simulink model "Robot"  (R2024b)
settings: Solver=ode4  StartTime=0.0  StopTime=inf  FixedStep=1/500  RelTol=1e-3  EnableMultiTasking=on
model workspace (MAT data in the model file):
  SL_ROS_VariableLengthArrays_MaxSizes.CommonInfo.ArrayTruncateAction = 'EmitWarning'
  SL_ROS_VariableLengthArrays_MaxSizes.MsgTypeMap = containers.Map
  SL_ROS_VariableLengthArrays_MaxSizes.MsgTypeMap.serialization.keys = {'trajectory_msgs/JointTrajectoryPoint'}
  SL_ROS_VariableLengthArrays_MaxSizes.MsgTypeMap.serialization.values{1}(1).PropertyName = 'accelerations'
  SL_ROS_VariableLengthArrays_MaxSizes.MsgTypeMap.serialization.values{1}(1).DataType = 'double'
  SL_ROS_VariableLengthArrays_MaxSizes.MsgTypeMap.serialization.values{1}(1).MaxLength = 4
  SL_ROS_VariableLengthArrays_MaxSizes.MsgTypeMap.serialization.values{1}(2).PropertyName = 'effort'
  SL_ROS_VariableLengthArrays_MaxSizes.MsgTypeMap.serialization.values{1}(2).DataType = 'double'
  SL_ROS_VariableLengthArrays_MaxSizes.MsgTypeMap.serialization.values{1}(2).MaxLength = 4
  SL_ROS_VariableLengthArrays_MaxSizes.MsgTypeMap.serialization.values{1}(3).PropertyName = 'positions'
  SL_ROS_VariableLengthArrays_MaxSizes.MsgTypeMap.serialization.values{1}(3).DataType = 'double'
  SL_ROS_VariableLengthArrays_MaxSizes.MsgTypeMap.serialization.values{1}(3).MaxLength = 5
  SL_ROS_VariableLengthArrays_MaxSizes.MsgTypeMap.serialization.values{1}(4).PropertyName = 'velocities'
  SL_ROS_VariableLengthArrays_MaxSizes.MsgTypeMap.serialization.values{1}(4).DataType = 'double'
  SL_ROS_VariableLengthArrays_MaxSizes.MsgTypeMap.serialization.values{1}(4).MaxLength = 4
  SL_ROS_VariableLengthArrays_MaxSizes.MsgTypeMap.serialization.uniformity = 0
  SL_ROS_VariableLengthArrays_MaxSizes.MsgTypeMap.serialization.keyType = 'char'
  SL_ROS_VariableLengthArrays_MaxSizes.MsgTypeMap.serialization.valueType = 'any'
undefined symbols (not defined in the file or in its folder): HIL, positions, positions_SL_Info
libraries: quarc_library x6, ros2lib x3
settings Model: ExtModeTrigDuration=10000  Creator=fvranes  LastModifiedBy=924287296
settings SolverCC: AlgebraicLoopSolver=TrustRegion  PositivePriorityOrder=on
settings DataIOCC: ReturnWorkspaceOutputs=off
settings OptimizationCC: DefaultParameterBehavior=Inlined  EnhancedBackFolding=on  PassReuseOutputArgsThreshold=0  MaxStackSize=64  OptimizeBlockOrder=speed  DifferentSizesBufferReuse=on  OptimizationCustomize=off
settings DebuggingCC: UnderspecifiedInitializationDetection=Classic  MergeDetectMultiDrivingBlocksExec=none  ParameterTunabilityLossMsg=error  UnconnectedInputMsg=warning  UnconnectedOutputMsg=warning  UnconnectedLineMsg=warning
settings ModelReferenceCC: EnableRefExpFcnMdlSchedulingChecks=on  PropagateSignalLabelsOutOfModel=off
settings SFSimCC: MATLABDynamicMemAlloc=off  CustomCodeUndefinedFunction=UseInterfaceOnly
settings RTWCC: Description=QUARC Win64 Target Using Toolchain  SystemTargetFile=quarc_win64.tlc  PackageGeneratedCodeAndArtifacts=on  TemplateMakefile=sldrt.tmf  Toolchain=QUARC win64 | nmake (64-bit Windows)  TargetLang=C++  GPUComputeCapability=3.5
settings RTWCC: CustomInclude=|
  | "Robot_ert_rtw"
  | "C:\Program Files\MATLAB\R2024b\sys\ros2\win64\ros2\include"
  | "C:\Program Files\MATLAB\R2024b\sys\ros2\win64\ros2\include\actionlib_msgs"
  | "C:\Program Files\MATLAB\R2024b\sys\ros2\win64\ros2\include\action_msgs"
  | "C:\Program Files\MATLAB\R2024b\sys\ros2\win64\ros2\include\action_tutorials_interfaces"
  | "C:\Program Files\MATLAB\R2024b\sys\ros2\win64\ros2\include\ament_index_cpp"
  | "C:\Program Files\MATLAB\R2024b\sys\ros2\win64\ros2\include\builtin_interfaces"
  | "C:\Program Files\MATLAB\R2024b\sys\ros2\win64\ros2\include\class_loader"
  | "C:\Program Files\MATLAB\R2024b\sys\ros2\win64\ros2\include\composition_interfaces"
  | "C:\Program Files\MATLAB\R2024b\sys\ros2\win64\ros2\include\console_bridge_vendor"
  | "C:\Program Files\MATLAB\R2024b\sys\ros2\win64\ros2\include\control_msgs"
  | "C:\Program Files\MATLAB\R2024b\sys\ros2\win64\ros2\include\dds"
  | "C:\Program Files\MATLAB\R2024b\sys\ros2\win64\ros2\include\ddsc"
  | "C:\Program Files\MATLAB\R2024b\sys\ros2\win64\ros2\include\diagnostic_msgs"
  | "C:\Program Files\MATLAB\R2024b\sys\ros2\win64\ros2\include\example_interfaces"
  | "C:\Program Files\MATLAB\R2024b\sys\ros2\win64\ros2\include\fastcdr"
  | "C:\Program Files\MATLAB\R2024b\sys\ros2\win64\ros2\include\fastdds"
  | "C:\Program Files\MATLAB\R2024b\sys\ros2\win64\ros2\include\fastrtps"
  | "C:\Program Files\MATLAB\R2024b\sys\ros2\win64\ros2\include\foonathan_memory"
  | "C:\Program Files\MATLAB\R2024b\sys\ros2\win64\ros2\include\geometry_msgs"
  | "C:\Program Files\MATLAB\R2024b\sys\ros2\win64\ros2\include\idl"
  | "C:\Program Files\MATLAB\R2024b\sys\ros2\win64\ros2\include\idlc"
  | "C:\Program Files\MATLAB\R2024b\sys\ros2\win64\ros2\include\keyboard_handler"
  | "C:\Program Files\MATLAB\R2024b\sys\ros2\win64\ros2\include\libstatistics_collector"
  | "C:\Program Files\MATLAB\R2024b\sys\ros2\win64\ros2\include\libyaml_vendor"
  | "C:\Program Files\MATLAB\R2024b\sys\ros2\win64\ros2\include\lifecycle_msgs"
  | "C:\Program Files\MATLAB\R2024b\sys\ros2\win64\ros2\include\logging_demo"
  | "C:\Program Files\MATLAB\R2024b\sys\ros2\win64\ros2\include\map_msgs"
  | "C:\Program Files\MATLAB\R2024b\sys\ros2\win64\ros2\include\mcap_vendor"
  | "C:\Program Files\MATLAB\R2024b\sys\ros2\win64\ros2\include\message_filters"
  | "C:\Program Files\MATLAB\R2024b\sys\ros2\win64\ros2\include\mimick"
  | "C:\Program Files\MATLAB\R2024b\sys\ros2\win64\ros2\include\moodycamel"
  | "C:\Program Files\MATLAB\R2024b\sys\ros2\win64\ros2\include\nav_msgs"
  | "C:\Program Files\MATLAB\R2024b\sys\ros2\win64\ros2\include\octomap_msgs"
  | "C:\Program Files\MATLAB\R2024b\sys\ros2\win64\ros2\include\pendulum_msgs"
  | "C:\Program Files\MATLAB\R2024b\sys\ros2\win64\ros2\include\pluginlib"
  | "C:\Program Files\MATLAB\R2024b\sys\ros2\win64\ros2\include\pybind11_vendor"
  | "C:\Program Files\MATLAB\R2024b\sys\ros2\win64\ros2\include\rcl"
  | "C:\Program Files\MATLAB\R2024b\sys\ros2\win64\ros2\include\rclcpp"
  | "C:\Program Files\MATLAB\R2024b\sys\ros2\win64\ros2\include\rclcpp_action"
  | "C:\Program Files\MATLAB\R2024b\sys\ros2\win64\ros2\include\rclcpp_components"
  | "C:\Program Files\MATLAB\R2024b\sys\ros2\win64\ros2\include\rclcpp_lifecycle"
  | "C:\Program Files\MATLAB\R2024b\sys\ros2\win64\ros2\include\rcl_action"
  | "C:\Program Files\MATLAB\R2024b\sys\ros2\win64\ros2\include\rcl_interfaces"
  | "C:\Program Files\MATLAB\R2024b\sys\ros2\win64\ros2\include\rcl_lifecycle"
  | "C:\Program Files\MATLAB\R2024b\sys\ros2\win64\ros2\include\rcl_logging_interface"
  | "C:\Program Files\MATLAB\R2024b\sys\ros2\win64\ros2\include\rcl_yaml_param_parser"
  | "C:\Program Files\MATLAB\R2024b\sys\ros2\win64\ros2\include\rcpputils"
  | "C:\Program Files\MATLAB\R2024b\sys\ros2\win64\ros2\include\rcutils"
  | "C:\Program Files\MATLAB\R2024b\sys\ros2\win64\ros2\include\rmw"
  | "C:\Program Files\MATLAB\R2024b\sys\ros2\win64\ros2\include\rmw_connextdds"
  | "C:\Program Files\MATLAB\R2024b\sys\ros2\win64\ros2\include\rmw_dds_common"
  | "C:\Program Files\MATLAB\R2024b\sys\ros2\win64\ros2\include\rmw_fastrtps_cpp"
  | "C:\Program Files\MATLAB\R2024b\sys\ros2\win64\ros2\include\rmw_fastrtps_dynamic_cpp"
  | "C:\Program Files\MATLAB\R2024b\sys\ros2\win64\ros2\include\rmw_fastrtps_shared_cpp"
  | "C:\Program Files\MATLAB\R2024b\sys\ros2\win64\ros2\include\ros2cli_test_interfaces"
  | "C:\Program Files\MATLAB\R2024b\sys\ros2\win64\ros2\include\rosbag2_compression"
  | "C:\Program Files\MATLAB\R2024b\sys\ros2\win64\ros2\include\rosbag2_compression_zstd"
  | "C:\Program Files\MATLAB\R2024b\sys\ros2\win64\ros2\include\rosbag2_cpp"
  | "C:\Program Files\MATLAB\R2024b\sys\ros2\win64\ros2\include\rosbag2_interfaces"
  | "C:\Program Files\MATLAB\R2024b\sys\ros2\win64\ros2\include\rosbag2_storage"
  | "C:\Program Files\MATLAB\R2024b\sys\ros2\win64\ros2\include\rosbag2_storage_default_plugins"
  | "C:\Program Files\MATLAB\R2024b\sys\ros2\win64\ros2\include\rosbag2_test_common"
  | "C:\Program Files\MATLAB\R2024b\sys\ros2\win64\ros2\include\rosbag2_transport"
  | "C:\Program Files\MATLAB\R2024b\sys\ros2\win64\ros2\include\rosgraph_msgs"
  | "C:\Program Files\MATLAB\R2024b\sys\ros2\win64\ros2\include\rosidl_runtime_c"
  | "C:\Program Files\MATLAB\R2024b\sys\ros2\win64\ros2\include\rosidl_runtime_cpp"
  | "C:\Program Files\MATLAB\R2024b\sys\ros2\win64\ros2\include\rosidl_typesupport_c"
  | "C:\Program Files\MATLAB\R2024b\sys\ros2\win64\ros2\include\rosidl_typesupport_cpp"
  | "C:\Program Files\MATLAB\R2024b\sys\ros2\win64\ros2\include\rosidl_typesupport_fastrtps_c"
  | "C:\Program Files\MATLAB\R2024b\sys\ros2\win64\ros2\include\rosidl_typesupport_fastrtps_cpp"
  | "C:\Program Files\MATLAB\R2024b\sys\ros2\win64\ros2\include\rosidl_typesupport_interface"
  | "C:\Program Files\MATLAB\R2024b\sys\ros2\win64\ros2\include\rosidl_typesupport_introspection_c"
  | "C:\Program Files\MATLAB\R2024b\sys\ros2\win64\ros2\include\rosidl_typesupport_introspection_cpp"
  | "C:\Program Files\MATLAB\R2024b\sys\ros2\win64\ros2\include\sensor_msgs"
  | "C:\Program Files\MATLAB\R2024b\sys\ros2\win64\ros2\include\shape_msgs"
  | "C:\Program Files\MATLAB\R2024b\sys\ros2\win64\ros2\include\spdlog"
  | "C:\Program Files\MATLAB\R2024b\sys\ros2\win64\ros2\include\statistics_msgs"
  | "C:\Program Files\MATLAB\R2024b\sys\ros2\win64\ros2\include\std_msgs"
  | "C:\Program Files\MATLAB\R2024b\sys\ros2\win64\ros2\include\std_srvs"
  | "C:\Program Files\MATLAB\R2024b\sys\ros2\win64\ros2\include\stereo_msgs"
  | "C:\Program Files\MATLAB\R2024b\sys\ros2\win64\ros2\include\test_msgs"
  | "C:\Program Files\MATLAB\R2024b\sys\ros2\win64\ros2\include\tf2"
  | "C:\Program Files\MATLAB\R2024b\sys\ros2\win64\ros2\include\tf2_msgs"
  | "C:\Program Files\MATLAB\R2024b\sys\ros2\win64\ros2\include\tf2_ros"
  | "C:\Program Files\MATLAB\R2024b\sys\ros2\win64\ros2\include\tracetools"
  | "C:\Program Files\MATLAB\R2024b\sys\ros2\win64\ros2\include\trajectory_msgs"
  | "C:\Program Files\MATLAB\R2024b\sys\ros2\win64\ros2\include\unique_identifier_msgs"
  | "C:\Program Files\MATLAB\R2024b\sys\ros2\win64\ros2\include\visualization_msgs"
  | "C:\Program Files\MATLAB\R2024b\toolbox\ros\slros2\src"
settings CodeAppCC: ForceParamTrailComments=on  MaxIdLength=95  OperatorAnnotations=on
settings STFCustomTargetCC: TargetLangStandard=C++20 (ISO)  ConcurrentExecutionCompliant=on  GRTInterface=on  UseToolchainInfoCompliant=on  SystemTargetFile=quarc_win64.tlc
settings GRTTargetCC: TargetLangStandard=C++20 (ISO)  ParMdlRefBuildCompliant=off  CompOptLevelCompliant=off  CombineOutputUpdateFcns=off  MatFileLogging=off  CPPClassGenCompliant=off  GRTInterface=on  ExtMode=on  ExtModeMexFile=quarc_comm

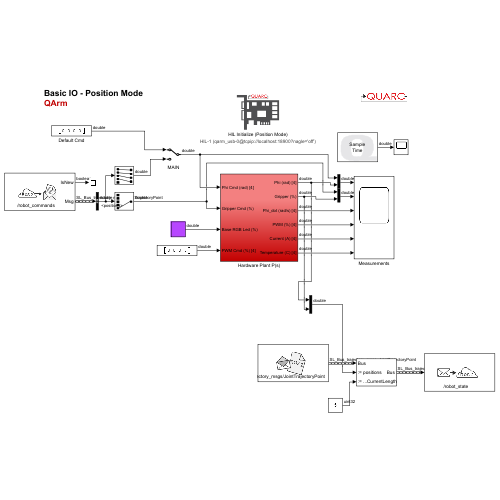
[thumbnail: Simulink's stored preview of the top-level diagram]
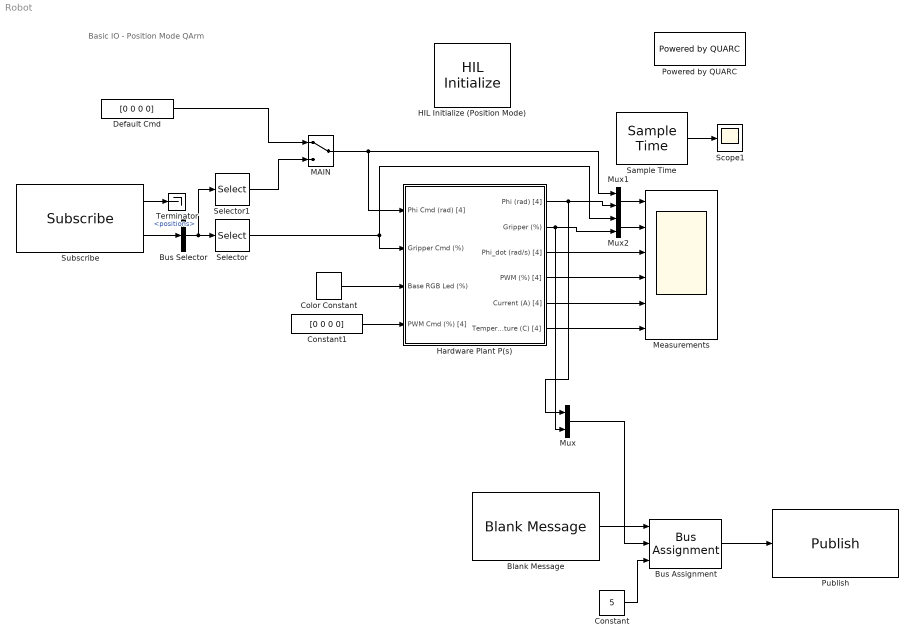
== system Robot ==
  note: Basic IO - Position Mode
      | QArm
  Blank Message : ros2lib/Blank Message  messageClass=Message  entityType=trajectory_msgs/JointTrajectoryPoint  messageType=trajectory_msgs/JointTrajectoryPoint  SampleTime=inf
  Bus Assignment : BusAssignment  AssignedSignals=positions,positions_SL_Info.CurrentLength
  Bus Selector : BusSelector  OutputSignals=positions
  Color Constant : quarc_library/Sources/Signals/Color Constant  color=[0.71765 0.27451 1]
      settings: SourceProductName=QUARC Targets
  Constant : Constant  Value=5  OutDataTypeStr=uint32
  Constant1 : Constant  Value=[0 0 0 0]
  Default Cmd : Constant  Value=[0 0 0 0]
  HIL Initialize (Position Mode) : quarc_library/Data Acquisition/Generic/Configuration/HIL Initialize  object_name=HIL-1  board_type=qarm_usb  board_number=0@tcpip://localhost:18900?nagle='off'  board_options=j0_mode=0;j1_mode=0;j2_mode=0;j3_mode=0;gripper_mode=0;  exclusive=off  active=on  hardware_clocks=[0]  clock_modes=[]  initial_clock_frequencies=[]  set_clock_params_at_start=off  set_clock_params_at_switch_in=off  set_clock_frequencies_at_start=off  set_clock_frequencies_at_switch_in=off  analog_input_channels=[5:9]  analog_input_configurations=[]  analog_input_maximums=[]  analog_input_minimums=[]  set_analog_input_params_at_start=off  set_analog_input_params_at_switch_in=off  analog_output_channels=[]  analog_output_maximums=inf  analog_output_minimums=-inf  initial_analog_outputs=[0]  final_analog_outputs=[0]  watchdog_analog_outputs=[]  set_analog_output_params_at_start=off  set_analog_output_params_at_switch_in=off  set_analog_outputs_at_start=off  set_analog_outputs_at_switch_in=off  set_analog_outputs_at_terminate=off  set_analog_outputs_at_switch_out=off  set_analog_outputs_on_watchdog=off  digital_input_channels=[]  digital_output_channels=[]  digital_output_configuration=[]  initial_digital_outputs=[0]  final_digital_outputs=[0]  watchdog_digital_outputs=[0]  set_digital_output_params_at_start=off  set_digital_output_params_at_switch_in=off  set_digital_outputs_at_start=off  set_digital_outputs_at_switch_in=off  set_digital_outputs_at_terminate=off  set_digital_outputs_at_switch_out=off  set_digital_outputs_on_watchdog=off  encoder_channels=[]  quadrature=[]  encoder_filter_frequency=[]  initial_encoder_counts=[]  set_encoder_params_at_start=off  set_encoder_params_at_switch_in=off  set_encoder_counts_at_start=off  set_encoder_counts_at_switch_in=off  pwm_channels=[]  pwm_modes=[]  pwm_frequency=[]  pwm_configuration=[]  pwm_alignment=[]  pwm_polarity=[]  pwm_leading_deadband=[]  pwm_trailing_deadband=[]  initial_pwm_outputs=[]  final_pwm_outputs=[]  watchdog_pwm_outputs=[]  set_pwm_params_at_start=off  set_pwm_params_at_switch_in=off  set_pwm_outputs_at_start=off  set_pwm_outputs_at_switch_in=off  set_pwm_outputs_at_terminate=off  set_pwm_outputs_at_switch_out=off  set_pwm_outputs_on_watchdog=off  other_output_channels=[1000:1004 11000:11003 11005:11007]  initial_other_outputs=[zeros(1,9), ones(1,3)]  final_other_outputs=[zeros(1,9), ones(1,3)]  watchdog_other_outputs=zeros(1,12)  set_other_outputs_at_start=off  set_other_outputs_at_switch_in=off  set_other_outputs_at_terminate=on  set_other_outputs_at_switch_out=off  set_other_outputs_on_watchdog=off
  Hardware Plant P(s) : Subsystem
  MAIN : ManualSwitch
  Measurements : Scope  NumInputPorts=6
  Mux : Mux  Inputs=2
  Mux1 : Mux  Inputs=2
  Mux2 : Mux  Inputs=2
  Powered by QUARC : quarc_library/Logos/Powered by QUARC
  Publish : ros2lib/Publish  topicSource=Select from ROS network  topic=/robot_state  messageType=trajectory_msgs/JointTrajectoryPoint  QOSHistory=Keep last  QOSDepth=1  QOSReliability=Reliable  QOSDurability=Volatile  QOSDeadline=Inf  QOSLifespan=Inf  QOSLiveliness=Automatic  QOSLeaseDuration=Inf  QOSAvoidROSNamespaceConventions=off
  Sample Time : quarc_library/Sources/Time/Sample Time  Priority=-99  sample_time=qc_get_step_size
  Scope1 : Scope
  Selector : Selector  InputPortWidth=5  IndexOptions=Index vector (dialog)  Indices=5  OutputSizes=1
  Selector1 : Selector  InputPortWidth=5  IndexOptions=Index vector (dialog)  Indices=1:4  OutputSizes=1
  Subscribe : ros2lib/Subscribe  topicSource=Select from ROS network  topic=/robot_commands  messageType=trajectory_msgs/JointTrajectoryPoint  sampleTime=-1  QOSHistory=Keep last  QOSDepth=1  QOSReliability=Reliable  QOSDurability=Volatile  QOSDeadline=Inf  QOSLifespan=Inf  QOSLiveliness=Automatic  QOSLeaseDuration=Inf  QOSAvoidROSNamespaceConventions=off
  Terminator : Terminator
  wires:
  Color Constant/1 -> Hardware Plant P(s)/3(Base RGB Led (%))
  Selector/1 -> Hardware Plant P(s)/2(Gripper Cmd (%)), Mux2/1
  Default Cmd/1 -> MAIN/1
  MAIN/1 -> Hardware Plant P(s)/1(Phi Cmd (rad) [4]), Mux1/1
  Hardware Plant P(s)/3(Phi_dot (rad/s) [4]) -> Measurements/3
  Hardware Plant P(s)/4(PWM (%) [4]) -> Measurements/4
  Hardware Plant P(s)/5(Current (A) [4]) -> Measurements/5
  Hardware Plant P(s)/6(Temperature (C) [4]) -> Measurements/6
  Mux1/1 -> Measurements/1
  Mux2/1 -> Measurements/2
  Hardware Plant P(s)/1(Phi (rad) [4]) -> Mux/1, Mux1/2
  Hardware Plant P(s)/2(Gripper (%)) -> Mux/2, Mux2/2
  Constant1/1 -> Hardware Plant P(s)/4(PWM Cmd (%) [4])
  Sample Time/1 -> Scope1/1
  Subscribe/2 -> Bus Selector/1
  Bus Selector/1 -> Selector1/1, Selector/1  "<positions>"
  Selector1/1 -> MAIN/2
  Blank Message/1 -> Bus Assignment/1
  Bus Assignment/1 -> Publish/1
  Mux/1 -> Bus Assignment/2
  Constant/1 -> Bus Assignment/3
  Subscribe/1 -> Terminator/1

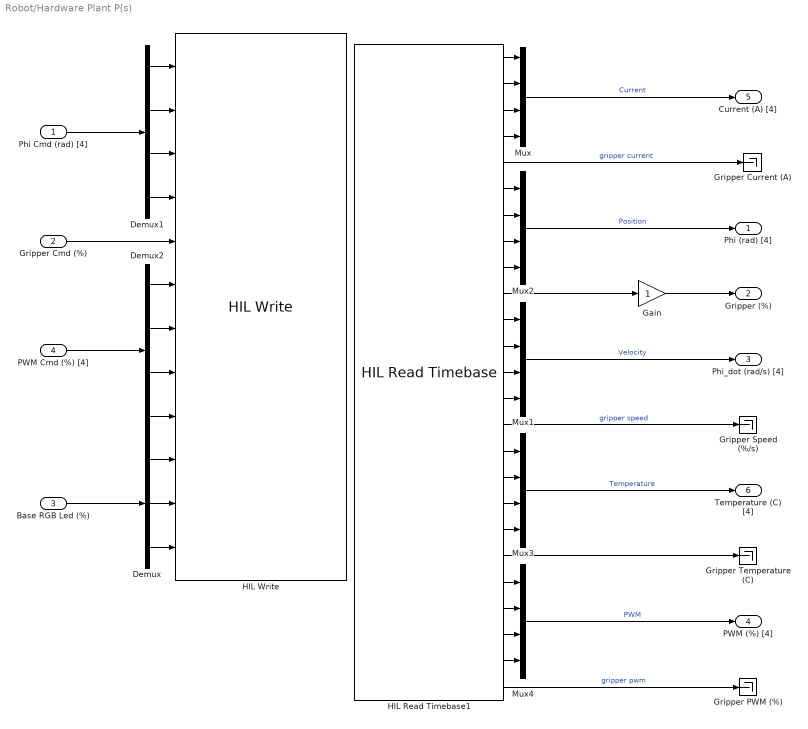
== system Robot/Hardware Plant P(s) ==
  Phi Cmd (rad) [4] : Inport
  Gripper Cmd (%) : Inport  Port=2
  Base RGB Led (%) : Inport  Port=3
  PWM Cmd (%) [4] : Inport  Port=4
  Demux : Demux  Outputs=3
  Demux1 : Demux
  Demux2 : Demux
  Gain : Gain
  Gripper Current (A) : Terminator
  Gripper PWM (%) : Terminator
  Gripper Speed (%/s) : Terminator
  Gripper Temperature (C) : Terminator
  HIL Read Timebase1 : quarc_library/Data Acquisition/Generic/Timebases/HIL Read Timebase  object_name=HIL-1  clock=0  analog_channels=[5:9]  encoder_channels=[]  digital_channels=[]  other_channels=[1000:1004 3000:3004 10000:10004 11000:11004]  active=on  vector_output=off  data_type_mode=Inherit via back propagation  encoder_data_type=double  digital_data_type=boolean  overflow_mode=Synchronize (for simulated cards only)  samples_in_buffer=1
  HIL Write : quarc_library/Data Acquisition/Generic/Immediate I//O/HIL Write  object_name=HIL-1  analog_channels=[]  pwm_channels=[]  digital_channels=[]  other_channels=[1000:1004 11000:11003 11005:11007]  sample_time=-1  active=on  vector_input=off
  Mux{,1..4} (5 alike) : Mux
  Phi (rad) [4] : Outport  VectorParamsAs1DForOutWhenUnconnected=off
  Gripper (%) : Outport  Port=2  VectorParamsAs1DForOutWhenUnconnected=off
  Phi_dot (rad/s) [4] : Outport  Port=3  VectorParamsAs1DForOutWhenUnconnected=off
  PWM (%) [4] : Outport  Port=4  VectorParamsAs1DForOutWhenUnconnected=off
  Current (A) [4] : Outport  Port=5  VectorParamsAs1DForOutWhenUnconnected=off
  Temperature (C) [4] : Outport  Port=6  VectorParamsAs1DForOutWhenUnconnected=off
  wires:
  Gripper Cmd (%)/1 -> HIL Write/5
  Gain/1 -> Gripper (%)/1
  HIL Read Timebase1/10 -> Gain/1
  Mux4/1 -> PWM (%) [4]/1  "PWM"
  HIL Read Timebase1/25 -> Gripper PWM (%)/1  "gripper pwm"
  HIL Read Timebase1/24 -> Mux4/4
  HIL Read Timebase1/23 -> Mux4/3
  HIL Read Timebase1/22 -> Mux4/2
  HIL Read Timebase1/21 -> Mux4/1
  Mux2/1 -> Phi (rad) [4]/1  "Position"
  Demux2/4 -> HIL Write/9
  Demux2/3 -> HIL Write/8
  Demux2/2 -> HIL Write/7
  Demux2/1 -> HIL Write/6
  PWM Cmd (%) [4]/1 -> Demux2/1
  Phi Cmd (rad) [4]/1 -> Demux1/1
  Demux1/4 -> HIL Write/4
  Demux1/3 -> HIL Write/3
  Demux1/2 -> HIL Write/2
  Demux1/1 -> HIL Write/1
  Base RGB Led (%)/1 -> Demux/1
  Mux3/1 -> Temperature (C) [4]/1  "Temperature"
  Mux1/1 -> Phi_dot (rad/s) [4]/1  "Velocity"
  Mux/1 -> Current (A) [4]/1  "Current"
  HIL Read Timebase1/20 -> Gripper Temperature (C)/1
  HIL Read Timebase1/1 -> Mux/1
  HIL Read Timebase1/2 -> Mux/2
  HIL Read Timebase1/13 -> Mux1/3
  Demux/2 -> HIL Write/11
  HIL Read Timebase1/19 -> Mux3/4
  Demux/1 -> HIL Write/10
  HIL Read Timebase1/11 -> Mux1/1
  HIL Read Timebase1/16 -> Mux3/1
  HIL Read Timebase1/17 -> Mux3/2
  HIL Read Timebase1/3 -> Mux/3
  Demux/3 -> HIL Write/12
  HIL Read Timebase1/15 -> Gripper Speed (%/s)/1  "gripper speed"
  HIL Read Timebase1/5 -> Gripper Current (A)/1  "gripper current"
  HIL Read Timebase1/7 -> Mux2/2
  HIL Read Timebase1/4 -> Mux/4
  HIL Read Timebase1/12 -> Mux1/2
  HIL Read Timebase1/8 -> Mux2/3
  HIL Read Timebase1/18 -> Mux3/3
  HIL Read Timebase1/6 -> Mux2/1
  HIL Read Timebase1/9 -> Mux2/4
  HIL Read Timebase1/14 -> Mux1/4
